simulink model "DalinovRegulatorNaDrugiNacin"  (R2013b)
settings: Solver=ode45  StartTime=0.0  StopTime=10.0  RelTol=1e-3
settings Model: Creator=Darko  LastModifiedBy=Darko

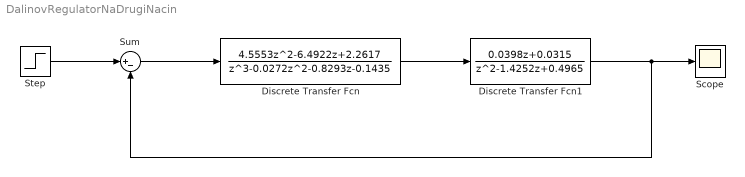
== system DalinovRegulatorNaDrugiNacin ==
  Discrete Transfer Fcn : DiscreteTransferFcn  Numerator=[4.5553 -6.4922 2.2617]  Denominator=[1 -0.0272 -0.8293 -0.1435]  SampleTime=0.1
  Discrete Transfer Fcn1 : DiscreteTransferFcn  Numerator=[0.0398 0.0315]  Denominator=[1 -1.4252 0.4965]  SampleTime=0.1
  Scope : Scope
  Step : Step  Time=0  SampleTime=0.01
  Sum : Sum  Inputs=|+-
  wires:
  Step/1 -> Sum/1
  Sum/1 -> Discrete Transfer Fcn/1
  Discrete Transfer Fcn/1 -> Discrete Transfer Fcn1/1
  Discrete Transfer Fcn1/1 -> Sum/2, Scope/1
